simulink model "NavigationProcessor"  (R2023b)
settings: Solver=VariableStepAuto  StartTime=0.0  StopTime=10.0  RelTol=1e-3
settings Model: Creator=user  LastModifiedBy=user

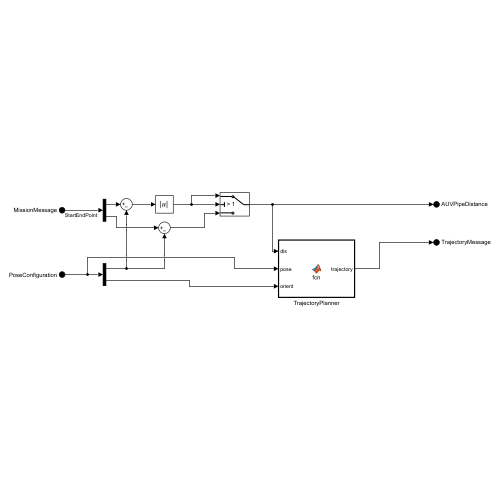
[thumbnail: Simulink's stored preview of the top-level diagram]
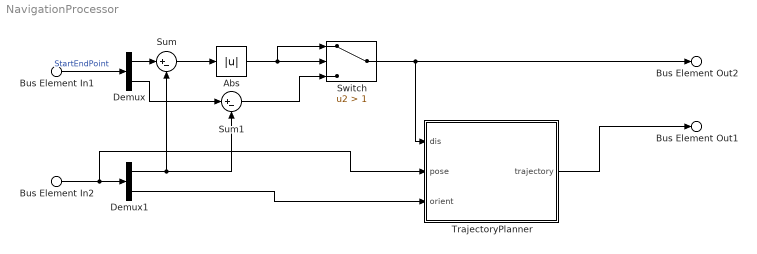
== system NavigationProcessor ==
  Bus Element In1 : Inport  PortName=MissionMessage
  Bus Element In2 : Inport  Port=2  PortName=PoseConfiguration
  Abs : Abs  SaturateOnIntegerOverflow=off
  Demux : Demux  Outputs=2
  Demux1 : Demux  Outputs=2
  Sum : Sum  Inputs=|+-
  Sum1 : Sum  Inputs=|+-
  Switch : Switch  Criteria=u2 > Threshold  Threshold=1  SaturateOnIntegerOverflow=off  InputSameDT=off
  TrajectoryPlanner : MATLAB Function  TreatAsAtomicUnit=on
  Bus Element Out1 : Outport  PortName=TrajectoryMessage
  Bus Element Out2 : Outport  Port=2  PortName=AUVPipeDistance
  wires:
  Bus Element In1/1 -> Demux/1  "StartEndPoint"
  Demux/1 -> Sum/1
  Sum/1 -> Abs/1
  Abs/1 -> Switch/1, Switch/2
  Demux/2 -> Sum1/1
  Sum1/1 -> Switch/3
  Switch/1 -> TrajectoryPlanner/1(dis), Bus Element Out2/1
  Bus Element In2/1 -> TrajectoryPlanner/2(pose), Demux1/1
  Demux1/1 -> Sum/2, Sum1/2
  TrajectoryPlanner/1(trajectory) -> Bus Element Out1/1
  Demux1/2 -> TrajectoryPlanner/3(orient)

== matlab function NavigationProcessor/TrajectoryPlanner ==
  data: dis input; trajectory output; pose input; orient input
function trajectory = fcn(dis, pose, orient)


u = 3*rand(2,1);

trajectory = u;
